simulink subsystem "LeastCov_v3_adaptiveAlgorithm"  (R2022a)
settings: Solver=VariableStepAuto  StartTime=0.0  StopTime=10.0  RelTol=1e-3
libraries: simulink x2, matrix_library x2
settings Model: Creator=targi  LastModifiedBy=targi

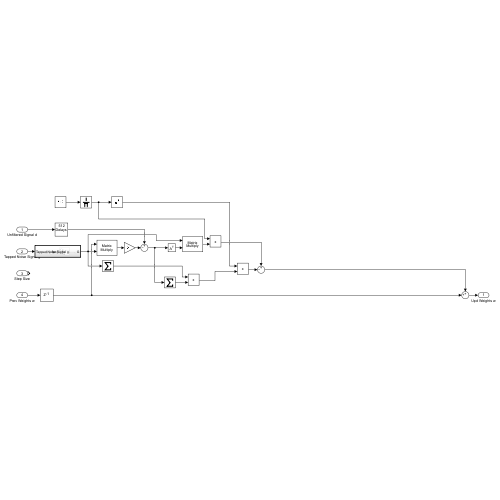
[thumbnail: Simulink's stored preview of the top-level diagram]
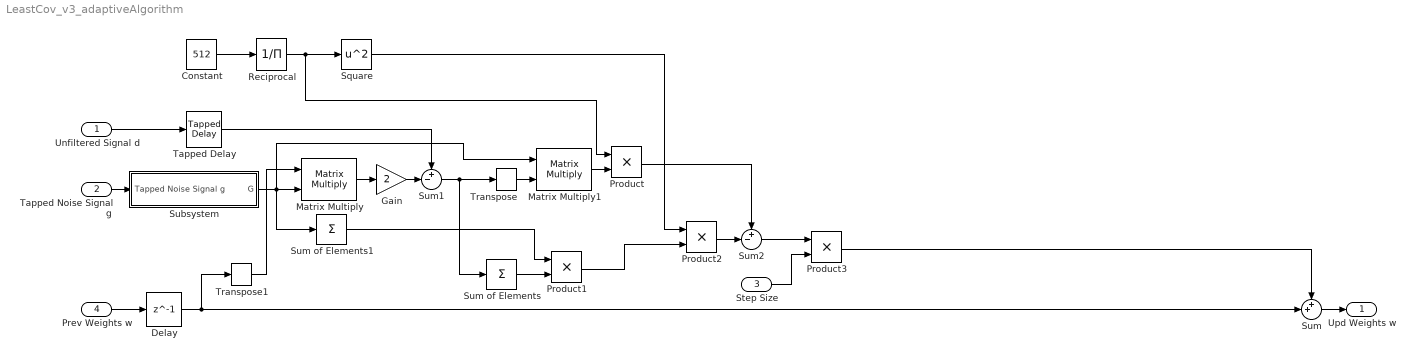
== system LeastCov_v3_adaptiveAlgorithm ==
  Unfiltered Signal d : Inport
  Tapped Noise Signal g : Inport  Port=2
  Step Size : Inport  Port=3
  Prev Weights w : Inport  Port=4
  Constant : Constant  Value=512
  Delay : Delay  DelayLength=1  InitialCondition=0
  Gain : Gain  Gain=2
  Matrix Multiply : Product  Multiplication=Matrix(*)
  Matrix Multiply1 : Product  Multiplication=Matrix(*)
  Product{,1..3} (4 alike) : Product
  Reciprocal : Product  Inputs=/
  Square : Math  Operator=square
  Subsystem : Subsystem
  Sum : Sum  Inputs=++|
  Sum of Elements : Sum  Inputs=+  CollapseMode=Specified dimension  CollapseDim=2
  Sum of Elements1 : Sum  Inputs=+  CollapseMode=Specified dimension  CollapseDim=2
  Sum1 : Sum  Inputs=+-|
  Sum2 : Sum  Inputs=+-|
  Tapped Delay : simulink/Discrete/Tapped Delay  vinit=0.0  samptime=-1  NumDelays=512  DelayOrder=Oldest  includeCurrent=off
  Transpose : matrix_library/Transpose
      settings: SourceProductBaseCode=SL
  Transpose1 : matrix_library/Transpose
      settings: SourceProductBaseCode=SL
  Upd Weights w : Outport
  wires:
  Product/1 -> Sum2/1
  Tapped Noise Signal g/1 -> Subsystem/1(Tapped Noise Signal g)
  Matrix Multiply1/1 -> Product/2
  Tapped Delay/1 -> Sum1/1
  Sum of Elements/1 -> Product1/2
  Sum/1 -> Upd Weights w/1
  Sum1/1 -> Sum of Elements/1, Transpose/1
  Square/1 -> Product2/1
  Product2/1 -> Sum2/2
  Constant/1 -> Reciprocal/1
  Reciprocal/1 -> Product/1, Square/1
  Product1/1 -> Product2/2
  Sum of Elements1/1 -> Product1/1
  Subsystem/1(G) -> Matrix Multiply1/1, Sum of Elements1/1, Matrix Multiply/2
  Prev Weights w/1 -> Delay/1
  Transpose/1 -> Matrix Multiply1/2
  Delay/1 -> Sum/2, Transpose1/1
  Gain/1 -> Sum1/2
  Unfiltered Signal d/1 -> Tapped Delay/1
  Matrix Multiply/1 -> Gain/1
  Transpose1/1 -> Matrix Multiply/1
  Sum2/1 -> Product3/1
  Step Size/1 -> Product3/2
  Product3/1 -> Sum/1

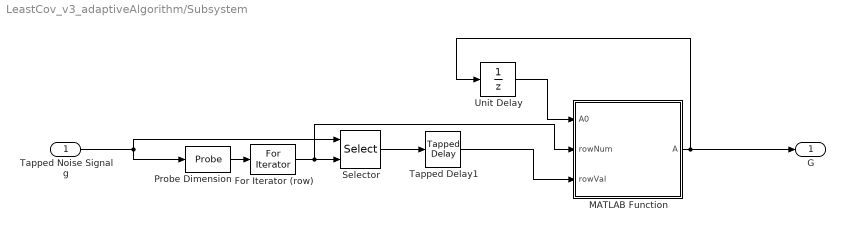
== system LeastCov_v3_adaptiveAlgorithm/Subsystem ==
  Tapped Noise Signal g : Inport
  For Iterator (row) : ForIterator  IterationSource=external
  MATLAB Function : MATLAB Function  TreatAsAtomicUnit=on
  Probe Dimension : Probe  ProbeSampleTime=off  ProbeComplexSignal=off
  Selector : Selector  IndexOptions=Starting index (port)  Indices=[1 3]  OutputSizes=1
  Tapped Delay1 : simulink/Discrete/Tapped Delay  vinit=0.0  samptime=-1  NumDelays=512  DelayOrder=Oldest  includeCurrent=off
  Unit Delay : UnitDelay  InitialCondition=zeros(256,512)  SampleTime=-1  HasFrameUpgradeWarning=on
  G : Outport
  wires:
  Unit Delay/1 -> MATLAB Function/1(A0)
  Tapped Delay1/1 -> MATLAB Function/3(rowVal)
  MATLAB Function/1(A) -> G/1, Unit Delay/1
  For Iterator (row)/1 -> Selector/2, MATLAB Function/2(rowNum)
  Probe Dimension/1 -> For Iterator (row)/1
  Tapped Noise Signal g/1 -> Selector/1, Probe Dimension/1
  Selector/1 -> Tapped Delay1/1

== matlab function LeastCov_v3_adaptiveAlgorithm/Subsystem/MATLAB Function ==
  data: A0 input; A output; rowNum input; rowVal input
function A = buildMatrix(A0, rowNum, rowVal)

A0(rowNum, :) = rowVal;
A = A0;
